simulink model "ekf"  (R2014b)
settings: Solver=ode45  StartTime=0.0  StopTime=65  RelTol=1e-3
values from neighbouring files (symbols this model uses):
  C1 = interp2(temp_array, voc_array, C1_array, initial_temp, initial_voc)    [load_sim_data.m]    (also in load_sim_data_v2.m; workspace.mat = 20030; workspace_2rc.mat = 181.78; workspace_comparison.mat = 181.78)
  C2 = interp2(temp_array, voc_array, C2_array, initial_temp, initial_voc)    [load_sim_data.m]    (also in load_sim_data_v2.m; workspace.mat = 33676.75; workspace_2rc.mat = 22.884; workspace_comparison.mat = 22.884)
  C_1 = 20030    [workspace.mat]
  C_2 = 33676.75    [workspace.mat]
  drive_profile = [0.003069801 0.003247245 0.003020715 0.003053892 0.002820143 0.003317081 0.003158873 0.002919445 0.002956375 0.002698265 0.002861501 0.002770798 ... (18750 elements, 1x18750)]    [drive_profile_ftp.mat]    (also in workspace.mat = [0 0 0 0 0 0 0 0 0 0 0 0 ... (521 elements, 1x521)]; workspace_2rc.mat; workspace_comparison.mat)
  drive_profile_index = [1 2 3 4 5 6 7 8 9 10 11 12 ... (18750 elements, 1x18750)]    [drive_profile_ftp.mat]    (also in load_sim_data_v2.m = drive_profile_index - 1; workspace.mat = [0 0.115384615385 0.230769230769 0.346153846154 0.4615384615; workspace_2rc.mat; workspace_comparison.mat)
  Q_total = 236.8    [load_sim_data.m]    (also in load_sim_data_v2.m = 350; workspace.mat = 44; workspace_2rc.mat = 44; workspace_comparison.mat = 44)
  R1 = interp2(temp_array, voc_array, R1_array, initial_temp, initial_voc)    [load_sim_data.m]    (also in load_sim_data_v2.m; workspace.mat = 0.00033425; workspace_2rc.mat = 0.0001483; workspace_comparison.mat = 0.0001483)
  R2 = interp2(temp_array, voc_array, R2_array, initial_temp, initial_voc)    [load_sim_data.m]    (also in load_sim_data_v2.m; workspace.mat = 0.000915125; workspace_2rc.mat = 0.0001594; workspace_comparison.mat = 0.0001594)
  R_1 = 0.00033425    [workspace.mat]
  R_2 = 0.000915125    [workspace.mat]
  R_i = 0.000736040625    [workspace.mat]
  Ri = interp2(temp_array, voc_array, Ri_array, initial_temp, initial_voc)    [load_sim_data.m]    (also in load_sim_data_v2.m; workspace.mat = 0.000736040625; workspace_2rc.mat = 0.0007932; workspace_comparison.mat = 0.0007932)
  T_gen = 0.1    [workspace.mat]
  Tgen = 1    [workspace.mat]    (also in workspace_2rc.mat; workspace_comparison.mat)
  Vmin = 3    [workspace.mat]    (also in workspace_2rc.mat; workspace_comparison.mat)
  voc_soc = [0 0.016393442623 0.0327868852459 0.0491803278689 0.0655737704918 0.0819672131148 0.0983606557377 0.114754098361 0.131147540984 0.147540983607 0.16393442623 0.180327868852 ... (124 elements, 62x2)]    [workspace.mat]
  voc_soc_lut = [3.07420931 3.44278771 3.51037487 3.58546258 3.63776945 3.68066188 3.73931818 3.84140797 3.94332291 4.0535654 4.18301283]    [emf_curve_single.mat]    (also in workspace.mat = [2.9985 3.0047 3.1504 3.2397 3.3026 3.3438 3.3699 3.3878 3.4; workspace_2rc.mat = [2.9985 3.0047 3.1504 3.2397 3.3026 3.3438 3.3699 3.3878 3.4; workspace_comparison.mat = [2.9985 3.0047 3.1504 3.2397 3.3026 3.3438 3.3699 3.3878 3.4)
  voc_soc_lut_index = [0 10 20 30 40 50 60 70 80 90 100]    [emf_curve_single.mat]    (also in workspace.mat = [0 1.6393442623 3.27868852459 4.91803278689 6.55737704918 8.; workspace_2rc.mat = [0 1.6393442623 3.27868852459 4.91803278689 6.55737704918 8.; workspace_comparison.mat = [0 1.6393442623 3.27868852459 4.91803278689 6.55737704918 8.)
libraries: fl_lib x11, nesl_utility x6
settings Model: Creator=OTG00077  LastModifiedBy=OTG00077

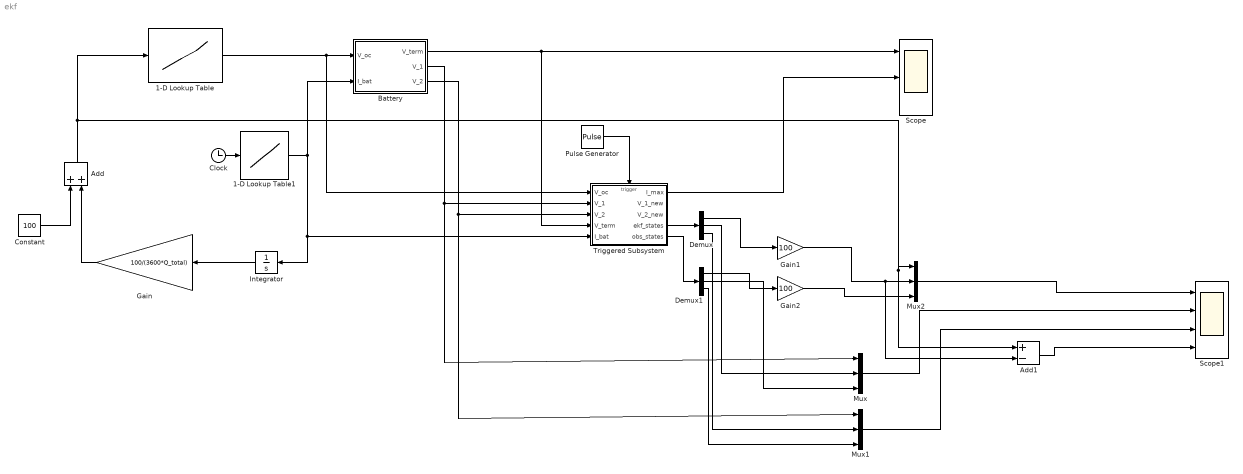
== system ekf ==
  1-D Lookup Table : Lookup_n-D  NumberOfTableDimensions=1  BreakpointsForDimension1=voc_soc_lut_index  Table=voc_soc_lut  InternalRulePriority=Speed  RndMeth=Simplest  InputSameDT=on
  1-D Lookup Table1 : Lookup_n-D  NumberOfTableDimensions=1  BreakpointsForDimension1=drive_profile_index  Table=drive_profile  InternalRulePriority=Speed  RndMeth=Simplest  InputSameDT=on
  Add : Sum
  Add1 : Sum  Inputs=+-
  Battery : Subsystem
  Clock : Clock
  Constant : Constant  Value=100
  Demux : Demux  Outputs=3
  Demux1 : Demux  Outputs=3
  Gain : Gain  Gain=100/(3600*Q_total)
  Gain1 : Gain  Gain=100
  Gain2 : Gain  Gain=100
  Integrator : Integrator
  Mux : Mux  Inputs=3
  Mux1 : Mux  Inputs=3
  Mux2 : Mux  Inputs=3
  Pulse Generator : DiscretePulseGenerator  PulseType=Time based  Period=T_gen  PulseWidth=5
  Scope : Scope  NumInputPorts=3
      settings: YMin=-5~-5~-5  YMax=5~5~5
  Scope1 : Scope  NumInputPorts=4
      settings: TimeRange=65  YMin=98.64576251147695~-0.015~-0.03~-20  YMax=99.45861169456775~0.005000000000000001~0.005000000000000004~100
  Triggered Subsystem : Subsystem  TreatAsAtomicUnit=on
  wires:
  Integrator/1 -> Gain/1
  Gain/1 -> Add/2
  Add/1 -> 1-D Lookup Table/1, Add1/1, Mux2/1
  Constant/1 -> Add/1
  Battery/2(V_1) -> Mux/1, Triggered Subsystem/2(V_1)
  Battery/3(V_2) -> Mux1/1, Triggered Subsystem/3(V_2)
  1-D Lookup Table/1 -> Triggered Subsystem/1(V_oc), Battery/1(V_oc)
  Pulse Generator/1 -> Triggered Subsystem/Trigger
  1-D Lookup Table1/1 -> Triggered Subsystem/5(I_bat), Integrator/1, Battery/2(I_bat)
  Clock/1 -> 1-D Lookup Table1/1
  Battery/1(V_term) -> Triggered Subsystem/4(V_term), Scope/1
  Triggered Subsystem/1(I_max) -> Scope/2
  Triggered Subsystem/4(ekf_states) -> Demux/1
  Demux/1 -> Gain1/1
  Gain1/1 -> Add1/2, Mux2/2
  Mux2/1 -> Scope1/1
  Demux/2 -> Mux/2
  Demux/3 -> Mux1/2
  Mux/1 -> Scope1/2
  Mux1/1 -> Scope1/3
  Add1/1 -> Scope1/4
  Triggered Subsystem/5(obs_states) -> Demux1/1
  Demux1/1 -> Gain2/1
  Gain2/1 -> Mux2/3
  Demux1/2 -> Mux/3
  Demux1/3 -> Mux1/3

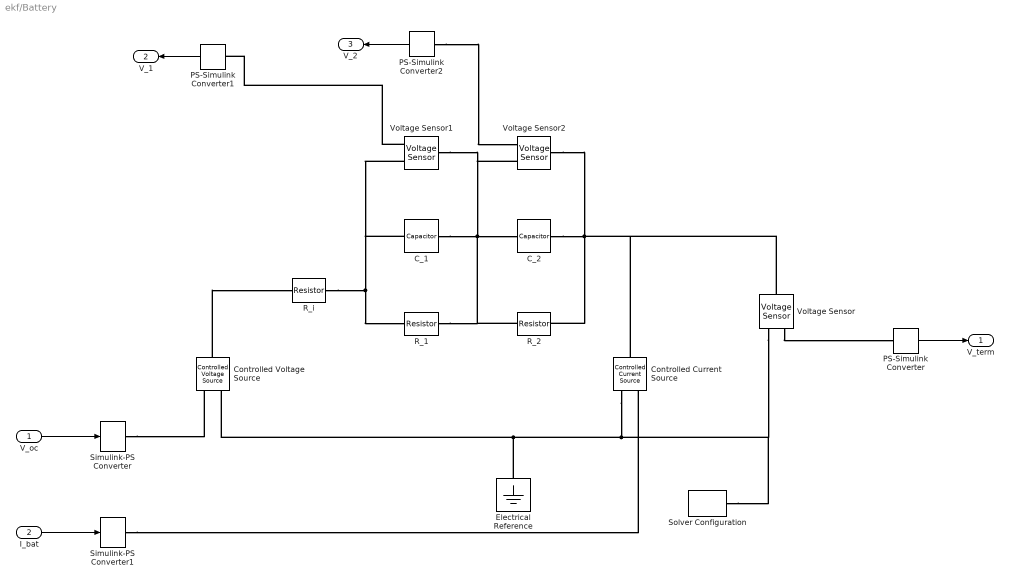
== system ekf/Battery ==
  V_oc : Inport
  I_bat : Inport  Port=2
  C_1 : fl_lib/Electrical/Electrical Elements/Capacitor  c=C1 F  r=0 Ohm  g=0 1/Ohm  i_specify=off  i_priority=High  i=0 A  v_specify=off  v_priority=High  v=0 V  vc_specify=off  vc_priority=High  vc=0 V
  C_2 : fl_lib/Electrical/Electrical Elements/Capacitor  c=C2 F  r=0 Ohm  g=0 1/Ohm  i_specify=off  i_priority=High  i=0 A  v_specify=off  v_priority=High  v=0 V  vc_specify=off  vc_priority=High  vc=0 V
  Controlled Current Source : fl_lib/Electrical/Electrical Sources/Controlled Current Source
  Controlled Voltage Source : fl_lib/Electrical/Electrical Sources/Controlled Voltage Source
  Electrical Reference : fl_lib/Electrical/Electrical Elements/Electrical Reference
  PS-Simulink Converter : nesl_utility/PS-Simulink Converter  PhysicalDomain=network_engine_domain  SubClassName=ps_output  LeftPortType=input  RightPortType=output  PseudoPeriodic=off  Frequencies=[]  Unit=1  AffineConversion=off
  PS-Simulink Converter1 : nesl_utility/PS-Simulink Converter  PhysicalDomain=network_engine_domain  SubClassName=ps_output  LeftPortType=input  RightPortType=output  PseudoPeriodic=off  Frequencies=[]  Unit=1  AffineConversion=off
  PS-Simulink Converter2 : nesl_utility/PS-Simulink Converter  PhysicalDomain=network_engine_domain  SubClassName=ps_output  LeftPortType=input  RightPortType=output  PseudoPeriodic=off  Frequencies=[]  Unit=1  AffineConversion=off
  R_1 : fl_lib/Electrical/Electrical Elements/Resistor  R=R1 Ohm  i_specify=off  i_priority=High  i=0 A  v_specify=off  v_priority=High  v=0 V
  R_2 : fl_lib/Electrical/Electrical Elements/Resistor  R=R2 Ohm  i_specify=off  i_priority=High  i=0 A  v_specify=off  v_priority=High  v=0 V
  R_i : fl_lib/Electrical/Electrical Elements/Resistor  R=3*Ri Ohm  i_specify=off  i_priority=High  i=0 A  v_specify=off  v_priority=High  v=0 V
  Simulink-PS Converter : nesl_utility/Simulink-PS Converter  PhysicalDomain=network_engine_domain  SubClassName=ps_input  LeftPortType=input  RightPortType=output  PseudoPeriodic=off  Frequencies=[]  NoiseDistribution=none  NoiseParameters=[]  Unit=1  AffineConversion=off  InputFiltering=off  SimscapeFilterOrder=1  InputFilterTimeConstant=0.001  UdotUserProvided=1
  Simulink-PS Converter1 : nesl_utility/Simulink-PS Converter  PhysicalDomain=network_engine_domain  SubClassName=ps_input  LeftPortType=input  RightPortType=output  PseudoPeriodic=off  Frequencies=[]  NoiseDistribution=none  NoiseParameters=[]  Unit=1  AffineConversion=off  InputFiltering=off  SimscapeFilterOrder=1  InputFilterTimeConstant=0.001  UdotUserProvided=1
  Solver Configuration : nesl_utility/Solver Configuration  PhysicalDomain=network_engine_domain  SubClassName=solver  LeftPortType=input  RightPortType=generic  Accelerate=off  Tones=[]  Harmonics=[]  SimulateNoise=off  Profile=off  UseLocalSampling=off  EnableSwitchedLinearOptims=on  FrequencyDomain=off  UseCCode=off  RelTol=0.001  AbsTol=1e-06  MinStep=1e-09  ToWorkspace=off  DoDC=off  ResidualTolerance=1e-09  UseLocalSolver=off  LocalSolverChoice=NE_BACKWARD_EULER_ADVANCER  LocalSolverSampleTime=0.001  DoFixedCost=off  MaxNonlinIter=3  MaxModeIter=2  LinearAlgebra=Sparse  DelaysMemoryBudget=1024  AutomaticFiltering=on  FilteringTimeConstant=0.001
  Voltage Sensor : fl_lib/Electrical/Electrical Sensors/Voltage Sensor
  Voltage Sensor1 : fl_lib/Electrical/Electrical Sensors/Voltage Sensor
  Voltage Sensor2 : fl_lib/Electrical/Electrical Sensors/Voltage Sensor
  V_term : Outport
  V_1 : Outport  Port=2
  V_2 : Outport  Port=3
  wires:
  V_oc/1 -> Simulink-PS Converter/1
  PS-Simulink Converter/1 -> V_term/1
  I_bat/1 -> Simulink-PS Converter1/1
  PS-Simulink Converter1/1 -> V_1/1
  PS-Simulink Converter2/1 -> V_2/1
  connections:
  R_i/RConn1 -- Voltage Sensor1/RConn2 -- C_1/LConn1 -- R_1/LConn1
  C_1/RConn1 -- Voltage Sensor2/RConn2 -- Voltage Sensor1/LConn1 -- R_2/LConn1 -- R_1/RConn1 -- C_2/LConn1
  C_2/RConn1 -- Voltage Sensor2/LConn1 -- R_2/RConn1 -- Controlled Current Source/LConn1 -- Voltage Sensor/LConn1
  Controlled Voltage Source/LConn1 -- R_i/LConn1
  Simulink-PS Converter/RConn1 -- Controlled Voltage Source/RConn1
  Voltage Sensor/RConn1 -- PS-Simulink Converter/LConn1
  Controlled Current Source/RConn2 -- Solver Configuration/RConn1 -- Voltage Sensor/RConn2 -- Electrical Reference/LConn1 -- Controlled Voltage Source/RConn2
  Simulink-PS Converter1/RConn1 -- Controlled Current Source/RConn1
  Voltage Sensor1/RConn1 -- PS-Simulink Converter1/LConn1
  PS-Simulink Converter2/LConn1 -- Voltage Sensor2/RConn1

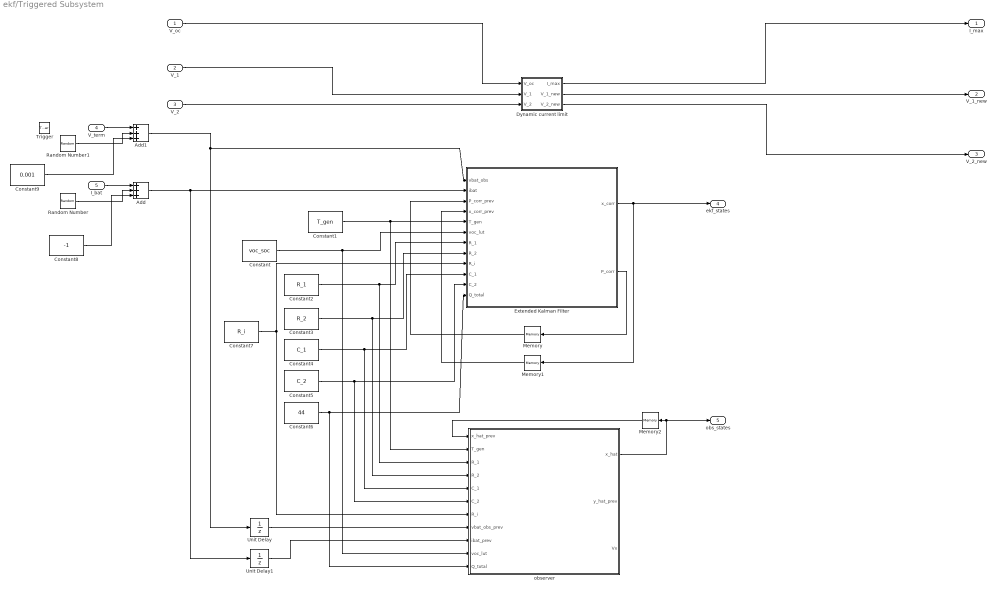
== system ekf/Triggered Subsystem ==
  V_oc : Inport
  V_1 : Inport  Port=2
  V_2 : Inport  Port=3
  V_term : Inport  Port=4
  I_bat : Inport  Port=5
  Trigger : TriggerPort
  Add : Sum  Inputs=+++
  Add1 : Sum  Inputs=+++
  Constant : Constant  Value=voc_soc
  Constant1 : Constant  Value=T_gen
  Constant2 : Constant  Value=R_1
  Constant3 : Constant  Value=R_2
  Constant4 : Constant  Value=C_1
  Constant5 : Constant  Value=C_2
  Constant6 : Constant  Value=44
  Constant7 : Constant  Value=R_i
  Constant8 : Constant  Value=-1
  Constant9 : Constant  Value=0.001
  Dynamic current limit : Subsystem
  Extended Kalman Filter : MATLAB Function  TreatAsAtomicUnit=on
  Memory : Memory  InheritSampleTime=on
  Memory1 : Memory  X0=[1; 0; 0]  InheritSampleTime=on
  Memory2 : Memory  X0=[1; 0; 0]  InheritSampleTime=on
  Random Number : RandomNumber  Variance=5
  Random Number1 : RandomNumber  Variance=0.01
  Unit Delay : UnitDelay  InitialCondition=4.1  SampleTime=-1
  Unit Delay1 : UnitDelay  SampleTime=-1
  observer : MATLAB Function  TreatAsAtomicUnit=on
  I_max : Outport
  V_1_new : Outport  Port=2
  V_2_new : Outport  Port=3
  ekf_states : Outport  Port=4
  obs_states : Outport  Port=5
  wires:
  V_oc/1 -> Dynamic current limit/1(V_oc)
  V_1/1 -> Dynamic current limit/2(V_1)
  V_2/1 -> Dynamic current limit/3(V_2)
  Dynamic current limit/1(I_max) -> I_max/1
  Dynamic current limit/2(V_1_new) -> V_1_new/1
  Dynamic current limit/3(V_2_new) -> V_2_new/1
  Constant/1 -> observer/10(voc_lut), Extended Kalman Filter/6(voc_lut)
  Constant1/1 -> observer/2(T_gen), Extended Kalman Filter/5(T_gen)
  Extended Kalman Filter/2(P_corr) -> Memory/1
  Extended Kalman Filter/1(x_corr) -> ekf_states/1, Memory1/1
  Memory/1 -> Extended Kalman Filter/3(P_corr_prev)
  Memory1/1 -> Extended Kalman Filter/4(x_corr_prev)
  Add1/1 -> Unit Delay/1, Extended Kalman Filter/1(vbat_obs)
  Add/1 -> Unit Delay1/1, Extended Kalman Filter/2(ibat)
  Constant2/1 -> observer/3(R_1), Extended Kalman Filter/7(R_1)
  Constant3/1 -> observer/4(R_2), Extended Kalman Filter/8(R_2)
  Constant4/1 -> observer/5(C_1), Extended Kalman Filter/10(C_1)
  Constant5/1 -> observer/6(C_2), Extended Kalman Filter/11(C_2)
  Constant6/1 -> observer/11(Q_total), Extended Kalman Filter/12(Q_total)
  Constant7/1 -> observer/7(R_i), Extended Kalman Filter/9(R_i)
  Unit Delay/1 -> observer/8(vbat_obs_prev)
  Unit Delay1/1 -> observer/9(ibat_prev)
  observer/1(x_hat) -> obs_states/1, Memory2/1
  Memory2/1 -> observer/1(x_hat_prev)
  Random Number/1 -> Add/2
  I_bat/1 -> Add/1
  Random Number1/1 -> Add1/2
  V_term/1 -> Add1/1
  Constant9/1 -> Add1/3
  Constant8/1 -> Add/3

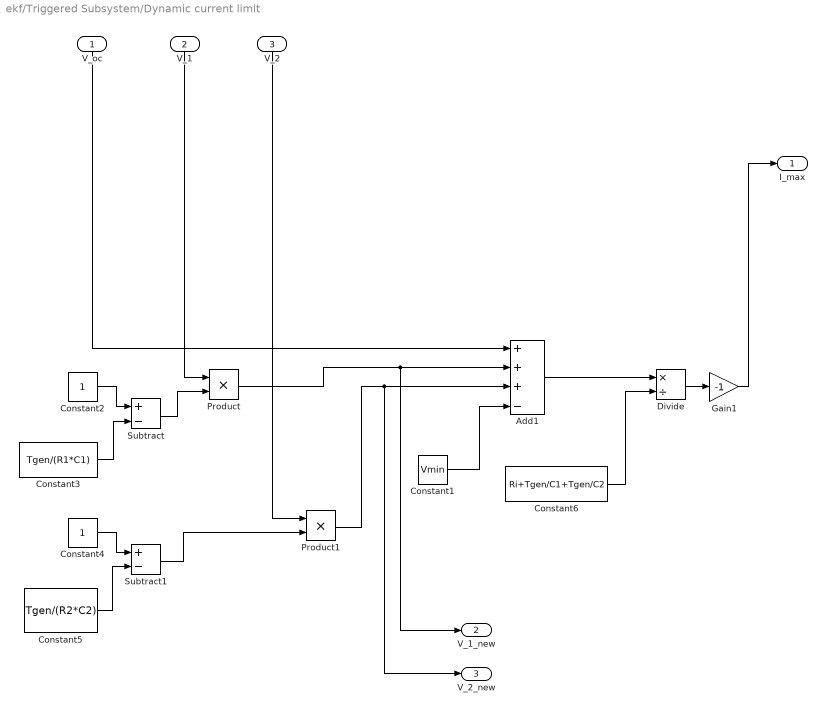
== system ekf/Triggered Subsystem/Dynamic current limit ==
  V_oc : Inport
  V_1 : Inport  Port=2
  V_2 : Inport  Port=3
  Add1 : Sum  Inputs=+++-
  Constant1 : Constant  Value=Vmin
  Constant2 : Constant
  Constant3 : Constant  Value=Tgen/(R1*C1)
  Constant4 : Constant
  Constant5 : Constant  Value=Tgen/(R2*C2)
  Constant6 : Constant  Value=Ri+Tgen/C1+Tgen/C2
  Divide : Product  Inputs=*/
  Gain1 : Gain  Gain=-1
  Product : Product
  Product1 : Product
  Subtract : Sum  Inputs=+-
  Subtract1 : Sum  Inputs=+-
  I_max : Outport
  V_1_new : Outport  Port=2
  V_2_new : Outport  Port=3
  wires:
  Constant5/1 -> Subtract1/2
  Constant2/1 -> Subtract/1
  V_1/1 -> Product/1
  V_2/1 -> Product1/1
  Subtract/1 -> Product/2
  Product/1 -> V_1_new/1, Add1/2
  Constant1/1 -> Add1/4
  Subtract1/1 -> Product1/2
  Divide/1 -> Gain1/1
  Constant3/1 -> Subtract/2
  V_oc/1 -> Add1/1
  Add1/1 -> Divide/1
  Product1/1 -> V_2_new/1, Add1/3
  Constant4/1 -> Subtract1/1
  Constant6/1 -> Divide/2
  Gain1/1 -> I_max/1

== matlab function ekf/Triggered Subsystem/observer ==
  data: x_hat_prev input size=[3,1]; x_hat output size=[3,1]; T_gen input; R_1 input; R_2 input; C_1 input; C_2 input; R_i input; vbat_obs_prev input; ibat_prev input; voc_lut input; Q_total input; y_hat_prev output; Vx output
function [x_hat,y_hat_prev,Vx] = obs(x_hat_prev, T_gen, R_1, R_2, C_1, C_2, R_i, vbat_obs_prev, ibat_prev, voc_lut, Q_total)
%#codegen

L=[0.000001; 0.000001;0.000001];

%A matrix
A=eye(3);
A(2,2)=1-T_gen/(R_1*C_1);
A(3,3)=1-T_gen/(R_2*C_2);

%B matrix
B=[100*T_gen/(3600*Q_total); T_gen/C_1; T_gen/C_2];

%calculate previous estimated output
index=1;
Vx=-1;
for i=1:length(voc_lut(:,1))
    if(x_hat_prev(1)==voc_lut(i,1))
        Vx=voc_lut(i,2);
    end
    if(x_hat_prev(1)>voc_lut(i,1))
        index=index+1;
    end
end

if(index<2)
    index=2;
elseif(index>62)
    index=62;
end
if (Vx==-1)
    Vx=(voc_lut(index,2)-voc_lut(index-1,2))/(voc_lut(index,1)-voc_lut(index-1,1))*(x_hat_prev(1)-voc_lut(index-1,1))+voc_lut(index-1,2);
end
    y_hat_prev=Vx+R_i*ibat_prev+x_hat_prev(2)+x_hat_prev(3);

%current state estimate
x_hat=A*x_hat_prev+B*ibat_prev+L*(vbat_obs_prev-y_hat_prev);
% A
% x_hat_prev
% B
% C
% L

== matlab function ekf/Triggered Subsystem/Extended Kalman Filter ==
  data: vbat_obs input; x_corr output size=[3,1]; ibat input; P_corr output size=[3,3]; P_corr_prev input size=[3,3]; x_corr_prev input size=[3,1]; T_gen input; voc_lut input; R_1 input; R_2 input; R_i input; C_1 input; C_2 input; Q_total input
function [x_corr, P_corr] = ekf(vbat_obs, ibat, P_corr_prev, x_corr_prev, T_gen, voc_lut, R_1, R_2, R_i, C_1, C_2, Q_total)
%#codegen

persistent x_pred P_pred;
if isempty(x_pred)
    x_pred=[1; 0; 0];
    P_pred=zeros(3);
end

sigma_ibat=5;
sigma_vbat=0.01;

%motion model jacobians
F=eye(3);
F(2,2)=1-T_gen/(R_1*C_1);
F(3,3)=1-T_gen/(R_2*C_2);

wprime=[T_gen/(3600*Q_total); T_gen/C_1; T_gen/C_2];

%prediction step
R=sigma_ibat^2;
Q=sigma_vbat^2;

P_pred=F*P_corr_prev*(F')+wprime*Q*(wprime');
x_pred=F*x_corr_prev+wprime*ibat;

%output model jacobians
index=1;
for i=1:length(voc_lut(:,1))
    if(x_pred(1)>=voc_lut(i,1))
        index=index+1;
    end
end
x_pred(1);

if(index<2)
    index=2;
elseif(index>62)
    index=62;
end
index;
m_oc=(voc_lut(index,2)-voc_lut(index-1,2))/(voc_lut(index,1)-voc_lut(index-1,1));
%voc_offset=voc_lut(index,2)+m_oc*((1+x_pred(1))-voc_lut(index,1))
voc_offset=voc_lut(index,2)-m_oc*x_pred(1);
G=[m_oc 1 1];

nprime=1;

%correction step
K=P_pred*(G')*(G*P_pred*(G')+nprime*R*(nprime'))^(-1);
P_corr=(eye(3)-K*G)*P_pred;
x_corr=x_pred+K*(vbat_obs-(G*x_pred+voc_offset+ibat*R_i));

P_pred
P_corr
x_corr
F
wprime*Q*(wprime')
nprime*R*(nprime')
G
K
